simulink model "frequency_count_v3"  (Simulink 10.1)
settings: Solver=ode45  StartTime=0.0  StopTime=2.5  FixedStep=5e-6  RelTol=1e-4  EnableMultiTasking=on
libraries: simulink x1
settings Model: Creator=mf  LastModifiedBy=Robin Vogt  ExtModeAutoUpdateStatusClock=off
settings DataIOCC: LimitDataPoints=on  SignalLoggingSaveFormat=ModelDataLogs  SignalLoggingName=sigsOut
settings OptimizationCC: BooleanDataType=off  ExpressionDepthLimit=2147483647
settings DebuggingCC: SaveWithParameterizedLinksMsg=none  SignalResolutionControl=TryResolveAllWithWarning  MultiTaskDSMMsg=warning  MultiTaskCondExecSysMsg=none  StateNameClashWarn=warning
settings HardwareCC: TargetUnknown=on
settings SFSimCC: SimParseCustomCode=off

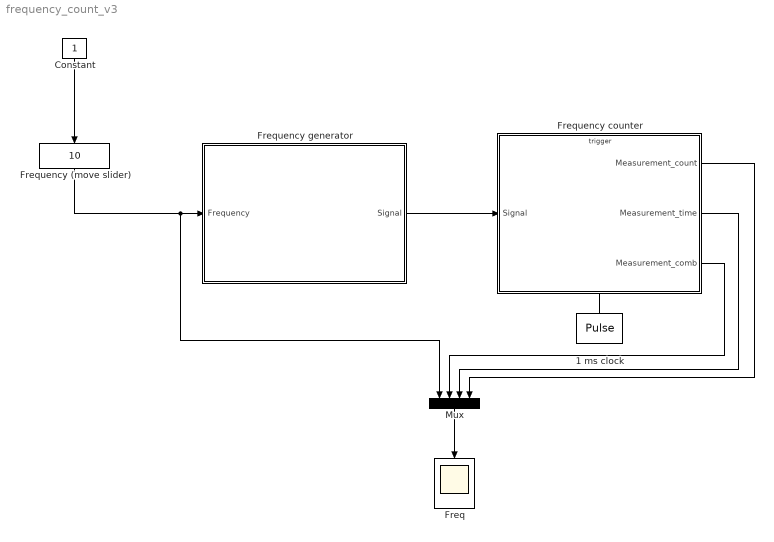
== system frequency_count_v3 ==
  1 ms clock : DiscretePulseGenerator  PulseType=Time based  Period=1e-3  PulseWidth=50
  Constant : Constant
  Freq : Scope
  Frequency (move slider) : simulink/Math Operations/Slider Gain  gain=10  low=1  high=500
  Frequency counter : Stateflow chart  TreatAsAtomicUnit=on
  Frequency generator : Subsystem
  Mux : Mux
  wires:
  Frequency generator/1(Signal) -> Frequency counter/1(Signal)
  Constant/1 -> Frequency (move slider)/1
  1 ms clock/1 -> Frequency counter/Trigger
  Mux/1 -> Freq/1
  Frequency (move slider)/1 -> Frequency generator/1(Frequency), Mux/1
  Frequency counter/1(Measurement_count) -> Mux/4
  Frequency counter/2(Measurement_time) -> Mux/3
  Frequency counter/3(Measurement_comb) -> Mux/2

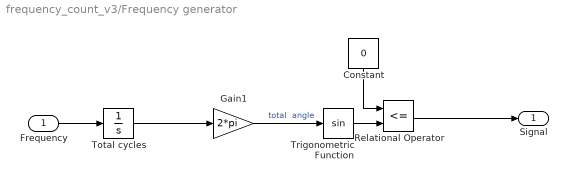
== system frequency_count_v3/Frequency generator ==
  Frequency : Inport
  Constant : Constant  Value=0
  Gain1 : Gain  Gain=2*pi  SaturateOnIntegerOverflow=on  OutDataTypeStr=Inherit: Same as input  ParamDataTypeStr=Inherit: Same as input
  Relational Operator : RelationalOperator  Operator=<=  OutDataTypeStr=boolean  RndMeth=Nearest
  Total cycles : Integrator
  Trigonometric Function : Trigonometry
  Signal : Outport
  wires:
  Frequency/1 -> Total cycles/1
  Trigonometric Function/1 -> Relational Operator/2
  Constant/1 -> Relational Operator/1
  Relational Operator/1 -> Signal/1
  Total cycles/1 -> Gain1/1
  Gain1/1 -> Trigonometric Function/1  "total  angle"

== stateflow chart Frequency counter ==
  settings: executeAtInitialization=1
  state FrequencyCounter
    state Measuring_Count [parallel]
      settings: executionOrder=2
      state Counter [parallel]
        settings: executionOrder=2
        state Initial_State
        state Signal_true
        state Signal_false
        (default) -> FrequencyCounter.Measuring_Count.Counter.Initial_State
        FrequencyCounter.Measuring_Count.Counter.Initial_State -> FrequencyCounter.Measuring_Count.Counter.Signal_true : [Signal]/{signal_count = 1;}
        FrequencyCounter.Measuring_Count.Counter.Signal_true -> FrequencyCounter.Measuring_Count.Counter.Signal_false : [~Signal]
        FrequencyCounter.Measuring_Count.Counter.Signal_false -> FrequencyCounter.Measuring_Count.Counter.Signal_true : [Signal]/{signal_count ++;}
      state Timer [parallel]
        settings: executionOrder=1
        state Clk_Counter/
          en:
          clk_count_c = 0;
          du:
          clk_count_c ++;
        (default) -> FrequencyCounter.Measuring_Count.Timer.Clk_Counter
        FrequencyCounter.Measuring_Count.Timer.Clk_Counter -> FrequencyCounter.Measuring_Count.Timer.Clk_Counter : [clk_count_c == time_interval_multiplier]/{
            | Measurement_count = (1000*signal_count)/time_interval_multiplier;
            | signal_count = 0;
            | clk_count_c = 0;}
    state Measuring_Time [parallel]
      settings: executionOrder=1
      state Initial_State
      state Signal_false
      state Signal_true
      (default) -> FrequencyCounter.Measuring_Time.Initial_State
      FrequencyCounter.Measuring_Time.Initial_State -> FrequencyCounter.Measuring_Time.Signal_true : [Signal]/{clk_count_t = 1;}
      FrequencyCounter.Measuring_Time.Signal_false -> FrequencyCounter.Measuring_Time.Signal_false [order 2] : {clk_count_t ++;}
      FrequencyCounter.Measuring_Time.Signal_true -> FrequencyCounter.Measuring_Time.Signal_true [order 2] : {clk_count_t ++;}
      FrequencyCounter.Measuring_Time.Signal_false -> FrequencyCounter.Measuring_Time.Signal_true [order 1] : [Signal]/{
          | Measurement_time = uint64(1000)/clk_count_t;
          | clk_count_t = 1;
          | }
      FrequencyCounter.Measuring_Time.Signal_true -> FrequencyCounter.Measuring_Time.Signal_false [order 1] : [~Signal]/{clk_count_t ++;}
    state Combination [parallel]
      settings: executionOrder=3
      state Timer [parallel]
        settings: executionOrder=2
        state Clk_Counter
        FrequencyCounter.Combination.Timer.Clk_Counter -> FrequencyCounter.Combination.Timer.Clk_Counter [order 2] : [signal_count_comb < signal_count_const]/{
            | clk_count_comb ++;}
        (default) -> FrequencyCounter.Combination.Timer.Clk_Counter
        FrequencyCounter.Combination.Timer.Clk_Counter -> FrequencyCounter.Combination.Timer.Clk_Counter [order 1] : [signal_count_comb == signal_count_const]/{
            | Measurement_comb = (1000*signal_count_comb)/clk_count_comb;
            | signal_count_comb = 0;
            | clk_count_comb = 0;}
      state Counter [parallel]
        settings: executionOrder=1
        state Initial_State
        state Signal_true
        state Signal_false
        (default) -> FrequencyCounter.Combination.Counter.Initial_State
        FrequencyCounter.Combination.Counter.Initial_State -> FrequencyCounter.Combination.Counter.Signal_true : [Signal]/{signal_count_comb = 1;}
        FrequencyCounter.Combination.Counter.Signal_true -> FrequencyCounter.Combination.Counter.Signal_false : [~Signal]
        FrequencyCounter.Combination.Counter.Signal_false -> FrequencyCounter.Combination.Counter.Signal_true : [Signal]/{signal_count_comb ++;}
  data: Signal input boolean; Measurement_count output double =0; signal_count local uint64 =uint64(0); Measurement_time output double =0; clk_count_c local uint64 =uint64(0); clk_count_t local uint64 =uint64(0); time_interval_multiplier constant uint8 =uint8(50); signal_count_const constant uint8 =10; clk_count_comb local uint64 =uint64(0); Measurement_comb output double; signal_count_comb local uint64 =uint64(0)
  events: clk input RISING_EDGE_EVENT
